simulink model "Realistic_scheme_2019"  (R2019b)
settings: Solver=VariableStepAuto  StartTime=0.0  StopTime=20  RelTol=1e-3
undefined symbols (not defined in the file or in its folder): A, B, C, Con_from_V, Con_to_V, D, K, Ts, V_max_in, V_max_out, wc
libraries: simulink x1
settings Model: Creator=elina  LastModifiedBy=gebruiker

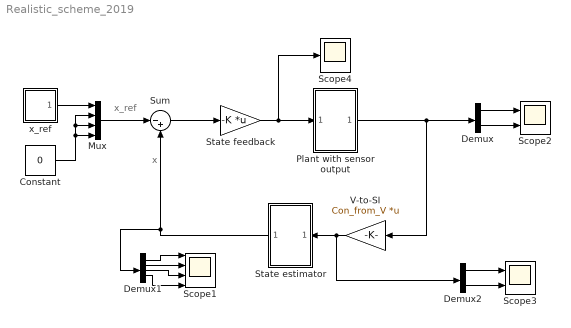
== system Realistic_scheme_2019 ==
  note: x_ref
  note: x
  Constant : Constant  Value=0
  Demux : Demux  Outputs=2
  Demux1 : Demux
  Demux2 : Demux  Outputs=2
  Mux : Mux
  Plant with sensor output : Subsystem
  Scope1 : Scope  NumInputPorts=4
  Scope2 : Scope  NumInputPorts=2
  Scope3 : Scope  NumInputPorts=2
  Scope4 : Scope
  State estimator : Subsystem
  State feedback : Gain  Gain=-K  Multiplication=Matrix(K*u)
  Sum : Sum  Inputs=|-+
  V-to-SI : Gain  Gain=Con_from_V  Multiplication=Matrix(K*u)
  x_ref : Subsystem
  wires:
  Sum/1 -> State feedback/1
  V-to-SI/1 -> Demux2/1, State estimator/1(In1)
  State feedback/1 -> Scope4/1, Plant with sensor output/1(In1)
  Constant/1 -> Mux/2, Mux/3, Mux/4
  State estimator/1(Out1) -> Demux1/1, Sum/2
  Mux/1 -> Sum/1
  x_ref/1(Out1) -> Mux/1
  Demux/1 -> Scope2/1
  Plant with sensor output/1(Out1) -> Demux/1, V-to-SI/1
  Demux/2 -> Scope2/2
  Demux1/1 -> Scope1/1
  Demux1/2 -> Scope1/2
  Demux1/3 -> Scope1/3
  Demux1/4 -> Scope1/4
  Demux2/1 -> Scope3/1
  Demux2/2 -> Scope3/2

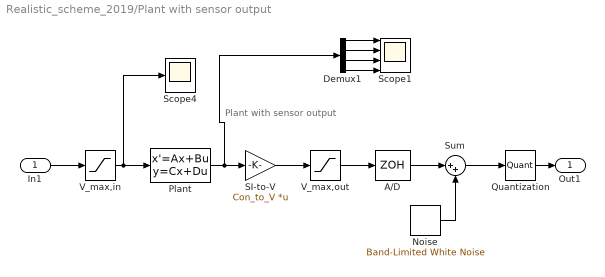
== system Realistic_scheme_2019/Plant with sensor output ==
  note: Plant with sensor output
  In1 : Inport
  A/D : ZeroOrderHold  SampleTime=Ts
  Demux1 : Demux
  Noise : simulink/Sources/Band-Limited White Noise  Cov=10e-10  Ts=Ts  seed=[23341]
  Plant : StateSpace  A=A  B=B  C=C  D=D  InitialCondition=[-0*0.5, 0*25*pi/180, 0, 0]
  Quantization : Quantizer  QuantizationInterval=quant_step
  SI-to-V : Gain  Gain=Con_to_V  Multiplication=Matrix(K*u)
  Scope1 : Scope  NumInputPorts=4
  Scope4 : Scope
  Sum : Sum  Inputs=|++
  V_max,in : Saturate  UpperLimit=V_max_in  LowerLimit=-V_max_in
  V_max,out : Saturate  UpperLimit=V_max_out  LowerLimit=-V_max_out
  Out1 : Outport
  wires:
  V_max,out/1 -> A/D/1
  SI-to-V/1 -> V_max,out/1
  Quantization/1 -> Out1/1
  A/D/1 -> Sum/1
  Sum/1 -> Quantization/1
  Noise/1 -> Sum/2
  In1/1 -> V_max,in/1
  V_max,in/1 -> Scope4/1, Plant/1
  Demux1/2 -> Scope1/2
  Demux1/1 -> Scope1/1
  Plant/1 -> Demux1/1, SI-to-V/1
  Demux1/3 -> Scope1/3
  Demux1/4 -> Scope1/4

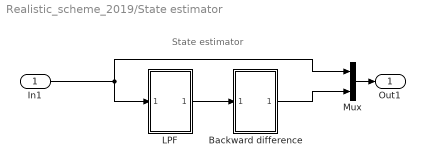
== system Realistic_scheme_2019/State estimator ==
  note: State estimator
  In1 : Inport
  Backward difference : Subsystem
  LPF : Subsystem
  Mux : Mux  Inputs=2
  Out1 : Outport
  wires:
  LPF/1(Out1) -> Backward difference/1(In1)
  Backward difference/1(Out1) -> Mux/2
  Mux/1 -> Out1/1
  In1/1 -> Mux/1, LPF/1(In1)

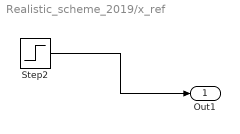
== system Realistic_scheme_2019/x_ref ==
  Step2 : Step  After=0.1  SampleTime=0
  Out1 : Outport
  wires:
  Step2/1 -> Out1/1

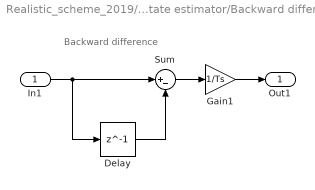
== system Realistic_scheme_2019/State estimator/Backward difference ==
  note: Backward difference
  In1 : Inport
  Delay : Delay  DelayLength=1  InitialCondition=0
  Gain1 : Gain  Gain=1/Ts
  Sum : Sum  Inputs=|+-
  Out1 : Outport
  wires:
  Delay/1 -> Sum/2
  Gain1/1 -> Out1/1
  In1/1 -> Delay/1, Sum/1
  Sum/1 -> Gain1/1

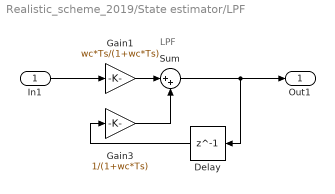
== system Realistic_scheme_2019/State estimator/LPF ==
  note: LPF
  In1 : Inport
  Delay : Delay  DelayLength=1
  Gain1 : Gain  Gain=wc*Ts/(1+wc*Ts)
  Gain3 : Gain  Gain=1/(1+wc*Ts)
  Sum : Sum  Inputs=|++
  Out1 : Outport
  wires:
  Gain3/1 -> Sum/2
  Sum/1 -> Out1/1, Delay/1
  Delay/1 -> Gain3/1
  In1/1 -> Gain1/1
  Gain1/1 -> Sum/1
